simulink model "SpinningMode"  (R2024b)
settings: configuration reference "STM32H7_Config" (kept outside this file)
undefined symbols (not defined in the file): MSpin, nRPMSpinningModelIntegralActivation, NSpinningModelKi, NSpinningModelKp, nTargetRPM, tSpinLength, tTorqueControlTask
libraries: simulink x3, simulink_extras x1
settings Model: DataDictionary=Master_Dictionary.sldd  EnableAccessToBaseWorkspace=off  Creator=torni  LastModifiedBy=William
settings ConfigSetRef: SourceName=STM32H7_Config

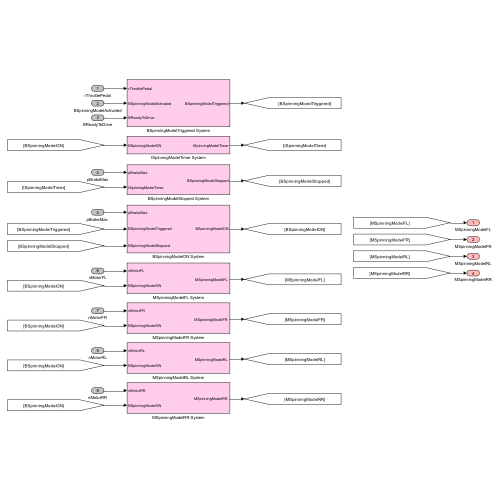
[thumbnail: Simulink's stored preview of the top-level diagram]
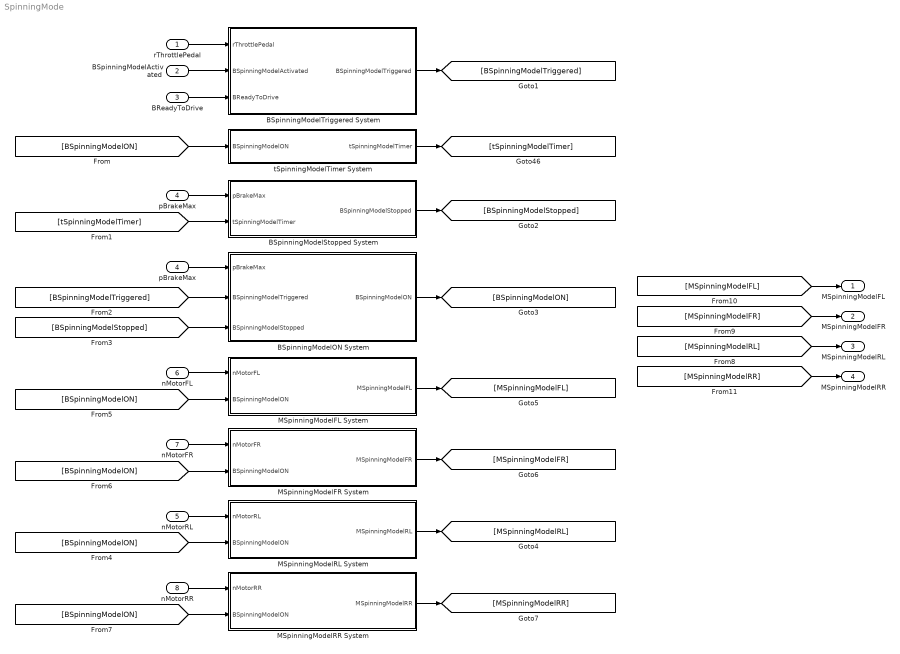
== system SpinningMode ==
  rThrottlePedal : Inport  OutDataTypeStr=double
  "BSpinningModelActivated " : Inport  Port=2  OutDataTypeStr=boolean
  BReadyToDrive : Inport  Port=3  OutDataTypeStr=boolean
  pBrakeMax : Inport  Port=4  OutDataTypeStr=double
  nMotorRL : Inport  Port=5  OutDataTypeStr=double
  nMotorFL : Inport  Port=6  OutDataTypeStr=double
  nMotorFR : Inport  Port=7  OutDataTypeStr=double
  nMotorRR : Inport  Port=8  OutDataTypeStr=double
  BSpinningModelON System : Subsystem
  BSpinningModelStopped System : Subsystem
  BSpinningModelTriggered System : Subsystem
  MSpinningModelFL System : Subsystem
  MSpinningModelFR System : Subsystem
  MSpinningModelRL System : Subsystem
  MSpinningModelRR System : Subsystem
  "pBrakeMax " : InportShadow  Port=4  OutDataTypeStr=double
  tSpinningModelTimer System : Subsystem
  MSpinningModelFL : Outport  OutDataTypeStr=double  VectorParamsAs1DForOutWhenUnconnected=off
  MSpinningModelFR : Outport  Port=2  OutDataTypeStr=double  VectorParamsAs1DForOutWhenUnconnected=off
  MSpinningModelRL : Outport  Port=3  OutDataTypeStr=double  VectorParamsAs1DForOutWhenUnconnected=off
  MSpinningModelRR : Outport  Port=4  OutDataTypeStr=double  VectorParamsAs1DForOutWhenUnconnected=off
  wires:
  rThrottlePedal/1 -> BSpinningModelTriggered System/1(rThrottlePedal)
  "BSpinningModelActivated "/1 -> BSpinningModelTriggered System/2("BSpinningModelActivated ")
  BReadyToDrive/1 -> BSpinningModelTriggered System/3(BReadyToDrive)
  pBrakeMax/1 -> BSpinningModelStopped System/1(pBrakeMax)
  [tSpinningModelTimer] -> BSpinningModelStopped System/2(tSpinningModelTimer)
  tSpinningModelTimer System/1(tSpinningModelTimer) -> [tSpinningModelTimer]
  BSpinningModelTriggered System/1(BSpinningModelTriggered) -> [BSpinningModelTriggered]
  BSpinningModelStopped System/1(BSpinningModelStopped) -> [BSpinningModelStopped]
  "pBrakeMax "/1 -> BSpinningModelON System/1(pBrakeMax)
  [BSpinningModelTriggered] -> BSpinningModelON System/2(BSpinningModelTriggered)
  [BSpinningModelStopped] -> BSpinningModelON System/3(BSpinningModelStopped)
  BSpinningModelON System/1(BSpinningModelON) -> [BSpinningModelON]
  [BSpinningModelON] -> tSpinningModelTimer System/1(BSpinningModelON)
  nMotorRL/1 -> MSpinningModelRL System/1(nMotorRL)
  [BSpinningModelON] -> MSpinningModelRL System/2(BSpinningModelON)
  MSpinningModelRL System/1("MSpinningModelRL ") -> [MSpinningModelRL]
  MSpinningModelFL System/1("MSpinningModelFL ") -> [MSpinningModelFL]
  [BSpinningModelON] -> MSpinningModelFL System/2(BSpinningModelON)
  nMotorFL/1 -> MSpinningModelFL System/1(nMotorFL)
  nMotorFR/1 -> MSpinningModelFR System/1(nMotorFR)
  [BSpinningModelON] -> MSpinningModelFR System/2(BSpinningModelON)
  MSpinningModelFR System/1("MSpinningModelFR ") -> [MSpinningModelFR]
  MSpinningModelRR System/1("MSpinningModelRR ") -> [MSpinningModelRR]
  [BSpinningModelON] -> MSpinningModelRR System/2(BSpinningModelON)
  nMotorRR/1 -> MSpinningModelRR System/1(nMotorRR)
  [MSpinningModelFL] -> MSpinningModelFL/1
  [MSpinningModelFR] -> MSpinningModelFR/1
  [MSpinningModelRR] -> MSpinningModelRR/1
  [MSpinningModelRL] -> MSpinningModelRL/1

== system SpinningMode/BSpinningModelON System ==
  pBrakeMax : Inport  OutDataTypeStr=double
  BSpinningModelTriggered : Inport  Port=2  OutDataTypeStr=boolean
  BSpinningModelStopped : Inport  Port=3  OutDataTypeStr=boolean
  Constant8 : Constant  Value=0
  S-R Flip-Flop : simulink_extras/Flip Flops/S-R Flip-Flop  initial_condition=0
  Switch3 : Switch  Criteria=u2 > Threshold  Threshold=1  SaturateOnIntegerOverflow=off  InputSameDT=off
  Terminator : Terminator
  BSpinningModelON : Outport  OutDataTypeStr=boolean  VectorParamsAs1DForOutWhenUnconnected=off
  wires:
  Switch3/1 -> BSpinningModelON/1
  BSpinningModelTriggered/1 -> S-R Flip-Flop/1
  Constant8/1 -> Switch3/1
  S-R Flip-Flop/1 -> Switch3/3
  S-R Flip-Flop/2 -> Terminator/1
  BSpinningModelStopped/1 -> S-R Flip-Flop/2
  pBrakeMax/1 -> Switch3/2

== system SpinningMode/BSpinningModelStopped System ==
  pBrakeMax : Inport  OutDataTypeStr=double
  tSpinningModelTimer : Inport  Port=2  OutDataTypeStr=double
  Compare To Constant : simulink/Logic and Bit Operations/Compare To Constant  relop=>  const=1  OutDataTypeStr=boolean
  Compare To Constant1 : simulink/Logic and Bit Operations/Compare To Constant  relop=>  const=tSpinLength  OutDataTypeStr=boolean
  OR1 : Logic  Operator=OR  AllPortsSameDT=off  OutDataTypeStr=boolean
  BSpinningModelStopped : Outport  OutDataTypeStr=boolean  VectorParamsAs1DForOutWhenUnconnected=off
  wires:
  Compare To Constant1/1 -> OR1/1
  Compare To Constant/1 -> OR1/2
  OR1/1 -> BSpinningModelStopped/1
  pBrakeMax/1 -> Compare To Constant/1
  tSpinningModelTimer/1 -> Compare To Constant1/1

== system SpinningMode/BSpinningModelTriggered System ==
  rThrottlePedal : Inport  OutDataTypeStr=double
  "BSpinningModelActivated " : Inport  Port=2  OutDataTypeStr=boolean
  BReadyToDrive : Inport  Port=3  OutDataTypeStr=boolean
  Compare To Constant : simulink/Logic and Bit Operations/Compare To Constant  relop=>  const=90  OutDataTypeStr=boolean
  Logical Operator : Logic  Inputs=3  AllPortsSameDT=off  OutDataTypeStr=boolean
  BSpinningModelTriggered : Outport  OutDataTypeStr=boolean  VectorParamsAs1DForOutWhenUnconnected=off
  wires:
  Logical Operator/1 -> BSpinningModelTriggered/1
  "BSpinningModelActivated "/1 -> Logical Operator/2
  rThrottlePedal/1 -> Compare To Constant/1
  Compare To Constant/1 -> Logical Operator/1
  BReadyToDrive/1 -> Logical Operator/3

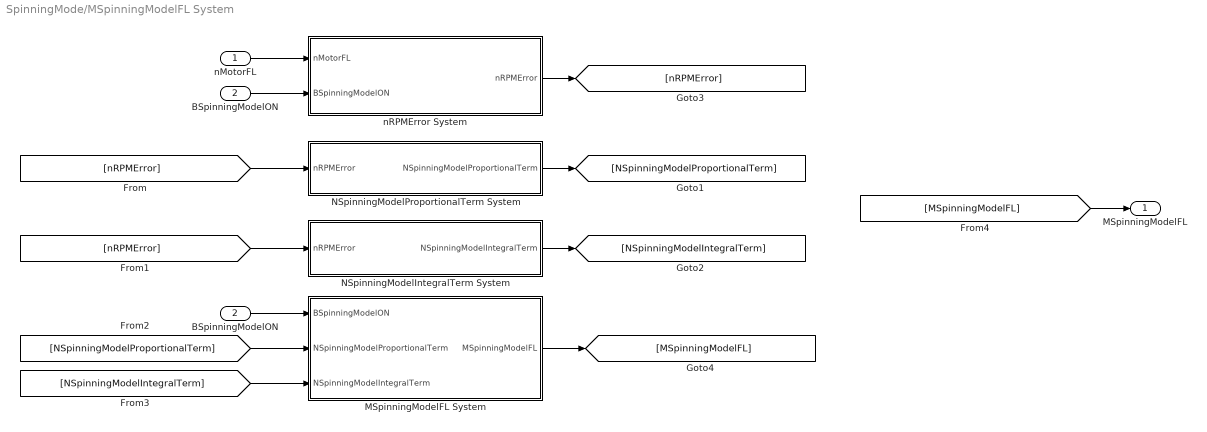
== system SpinningMode/MSpinningModelFL System ==
  nMotorFL : Inport  OutDataTypeStr=double
  BSpinningModelON : Inport  Port=2  OutDataTypeStr=boolean
  "BSpinningModelON " : InportShadow  Port=2  OutDataTypeStr=boolean
  MSpinningModelFL System : Subsystem
  NSpinningModelIntegralTerm System : Subsystem
  NSpinningModelProportionalTerm System : Subsystem
  nRPMError System : Subsystem
  "MSpinningModelFL " : Outport  OutDataTypeStr=double  VectorParamsAs1DForOutWhenUnconnected=off
  wires:
  [MSpinningModelFL] -> "MSpinningModelFL "/1
  MSpinningModelFL System/1("MSpinningModelFL ") -> [MSpinningModelFL]
  "BSpinningModelON "/1 -> MSpinningModelFL System/1(BSpinningModelON)
  [NSpinningModelIntegralTerm] -> MSpinningModelFL System/3(NSpinningModelIntegralTerm)
  [NSpinningModelProportionalTerm] -> MSpinningModelFL System/2(NSpinningModelProportionalTerm)
  NSpinningModelIntegralTerm System/1(NSpinningModelIntegralTerm) -> [NSpinningModelIntegralTerm]
  [nRPMError] -> NSpinningModelIntegralTerm System/1(nRPMError)
  NSpinningModelProportionalTerm System/1(NSpinningModelProportionalTerm) -> [NSpinningModelProportionalTerm]
  [nRPMError] -> NSpinningModelProportionalTerm System/1(nRPMError)
  nRPMError System/1(nRPMError) -> [nRPMError]
  BSpinningModelON/1 -> nRPMError System/2(BSpinningModelON)
  nMotorFL/1 -> nRPMError System/1(nMotorFL)

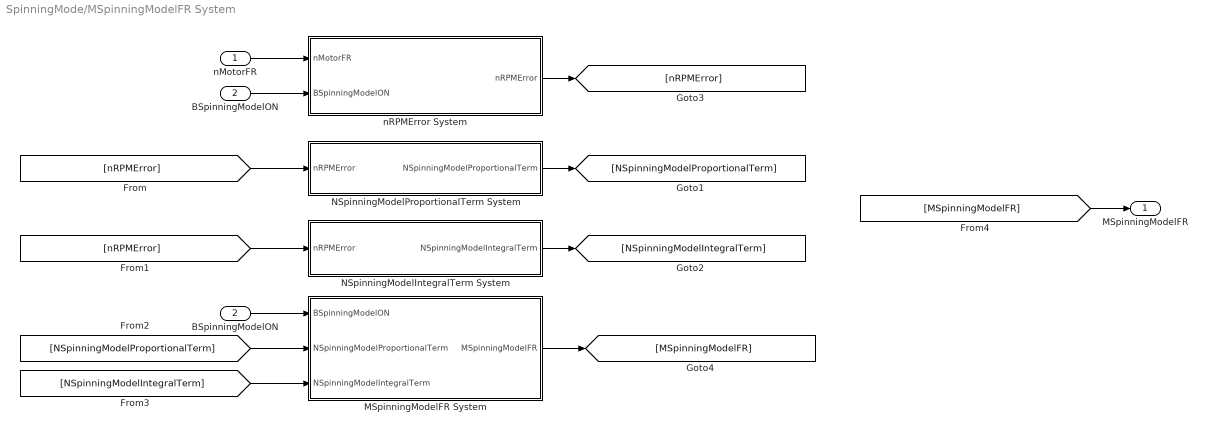
== system SpinningMode/MSpinningModelFR System ==
  nMotorFR : Inport  OutDataTypeStr=double
  BSpinningModelON : Inport  Port=2  OutDataTypeStr=boolean
  "BSpinningModelON " : InportShadow  Port=2  OutDataTypeStr=boolean
  MSpinningModelFR System : Subsystem
  NSpinningModelIntegralTerm System : Subsystem
  NSpinningModelProportionalTerm System : Subsystem
  nRPMError System : Subsystem
  "MSpinningModelFR " : Outport  OutDataTypeStr=double  VectorParamsAs1DForOutWhenUnconnected=off
  wires:
  nMotorFR/1 -> nRPMError System/1(nMotorFR)
  BSpinningModelON/1 -> nRPMError System/2(BSpinningModelON)
  nRPMError System/1(nRPMError) -> [nRPMError]
  [nRPMError] -> NSpinningModelProportionalTerm System/1(nRPMError)
  NSpinningModelProportionalTerm System/1(NSpinningModelProportionalTerm) -> [NSpinningModelProportionalTerm]
  [nRPMError] -> NSpinningModelIntegralTerm System/1(nRPMError)
  NSpinningModelIntegralTerm System/1(NSpinningModelIntegralTerm) -> [NSpinningModelIntegralTerm]
  [NSpinningModelProportionalTerm] -> MSpinningModelFR System/2(NSpinningModelProportionalTerm)
  [NSpinningModelIntegralTerm] -> MSpinningModelFR System/3(NSpinningModelIntegralTerm)
  "BSpinningModelON "/1 -> MSpinningModelFR System/1(BSpinningModelON)
  MSpinningModelFR System/1("MSpinningModelFR ") -> [MSpinningModelFR]
  [MSpinningModelFR] -> "MSpinningModelFR "/1

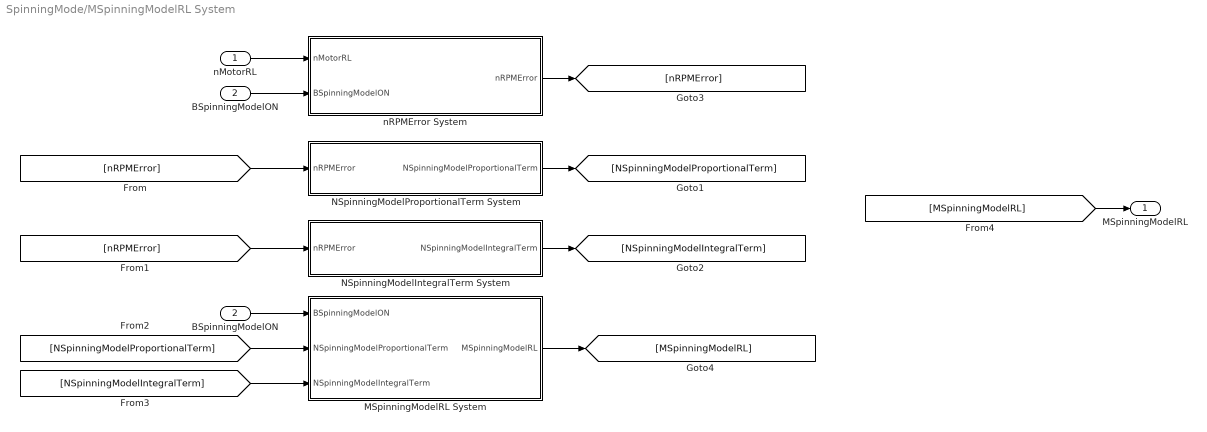
== system SpinningMode/MSpinningModelRL System ==
  nMotorRL : Inport  OutDataTypeStr=double
  BSpinningModelON : Inport  Port=2  OutDataTypeStr=boolean
  "BSpinningModelON " : InportShadow  Port=2  OutDataTypeStr=boolean
  MSpinningModelRL System : Subsystem
  NSpinningModelIntegralTerm System : Subsystem
  NSpinningModelProportionalTerm System : Subsystem
  nRPMError System : Subsystem
  "MSpinningModelRL " : Outport  OutDataTypeStr=double  VectorParamsAs1DForOutWhenUnconnected=off
  wires:
  nMotorRL/1 -> nRPMError System/1(nMotorRL)
  BSpinningModelON/1 -> nRPMError System/2(BSpinningModelON)
  nRPMError System/1(nRPMError) -> [nRPMError]
  [nRPMError] -> NSpinningModelProportionalTerm System/1(nRPMError)
  NSpinningModelProportionalTerm System/1(NSpinningModelProportionalTerm) -> [NSpinningModelProportionalTerm]
  [nRPMError] -> NSpinningModelIntegralTerm System/1(nRPMError)
  NSpinningModelIntegralTerm System/1(NSpinningModelIntegralTerm) -> [NSpinningModelIntegralTerm]
  [NSpinningModelProportionalTerm] -> MSpinningModelRL System/2(NSpinningModelProportionalTerm)
  [NSpinningModelIntegralTerm] -> MSpinningModelRL System/3(NSpinningModelIntegralTerm)
  "BSpinningModelON "/1 -> MSpinningModelRL System/1(BSpinningModelON)
  MSpinningModelRL System/1("MSpinningModelRL ") -> [MSpinningModelRL]
  [MSpinningModelRL] -> "MSpinningModelRL "/1

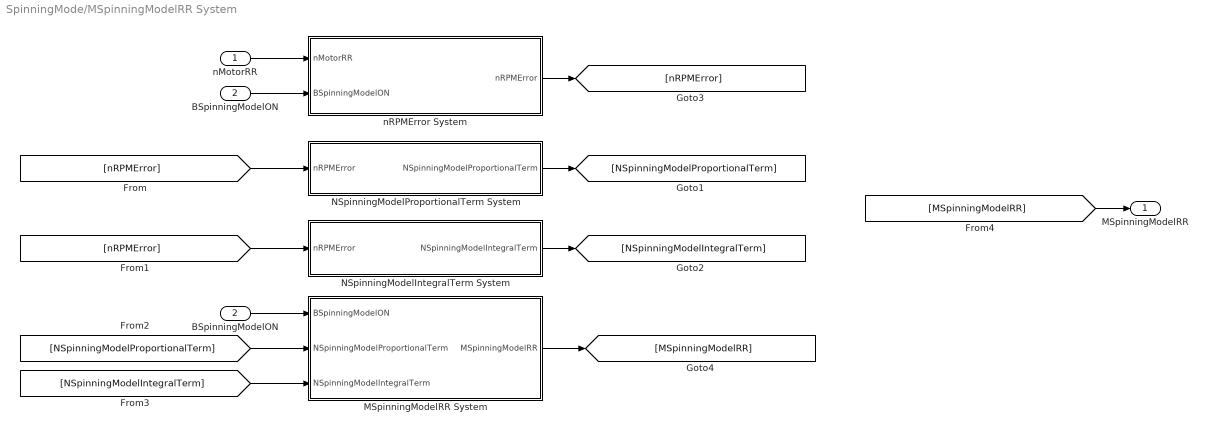
== system SpinningMode/MSpinningModelRR System ==
  nMotorRR : Inport  OutDataTypeStr=double
  BSpinningModelON : Inport  Port=2  OutDataTypeStr=boolean
  "BSpinningModelON " : InportShadow  Port=2  OutDataTypeStr=boolean
  MSpinningModelRR System : Subsystem
  NSpinningModelIntegralTerm System : Subsystem
  NSpinningModelProportionalTerm System : Subsystem
  nRPMError System : Subsystem
  "MSpinningModelRR " : Outport  OutDataTypeStr=double  VectorParamsAs1DForOutWhenUnconnected=off
  wires:
  [MSpinningModelRR] -> "MSpinningModelRR "/1
  MSpinningModelRR System/1("MSpinningModelRR ") -> [MSpinningModelRR]
  "BSpinningModelON "/1 -> MSpinningModelRR System/1(BSpinningModelON)
  [NSpinningModelIntegralTerm] -> MSpinningModelRR System/3(NSpinningModelIntegralTerm)
  [NSpinningModelProportionalTerm] -> MSpinningModelRR System/2(NSpinningModelProportionalTerm)
  NSpinningModelIntegralTerm System/1(NSpinningModelIntegralTerm) -> [NSpinningModelIntegralTerm]
  [nRPMError] -> NSpinningModelIntegralTerm System/1(nRPMError)
  NSpinningModelProportionalTerm System/1(NSpinningModelProportionalTerm) -> [NSpinningModelProportionalTerm]
  [nRPMError] -> NSpinningModelProportionalTerm System/1(nRPMError)
  nRPMError System/1(nRPMError) -> [nRPMError]
  BSpinningModelON/1 -> nRPMError System/2(BSpinningModelON)
  nMotorRR/1 -> nRPMError System/1(nMotorRR)

== system SpinningMode/tSpinningModelTimer System ==
  BSpinningModelON : Inport  OutDataTypeStr=boolean
  Add1 : Sum
  Constant5 : Constant  Value=tTorqueControlTask
  Constant6 : Constant  Value=0
  Memory1 : Memory  InheritSampleTime=on
  Switch1 : Switch  Criteria=u2 > Threshold  Threshold=0.5  SaturateOnIntegerOverflow=off  InputSameDT=off
  tSpinningModelTimer : Outport  OutDataTypeStr=double  VectorParamsAs1DForOutWhenUnconnected=off
  wires:
  Add1/1 -> Memory1/1
  Memory1/1 -> tSpinningModelTimer/1, Switch1/1
  Switch1/1 -> Add1/1
  Constant5/1 -> Add1/2
  Constant6/1 -> Switch1/3
  BSpinningModelON/1 -> Switch1/2

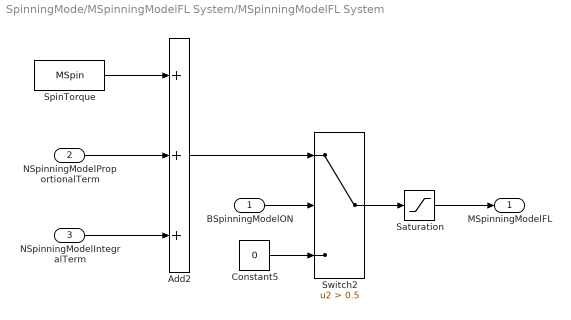
== system SpinningMode/MSpinningModelFL System/MSpinningModelFL System ==
  BSpinningModelON : Inport  OutDataTypeStr=boolean
  NSpinningModelProportionalTerm : Inport  Port=2  OutDataTypeStr=double
  NSpinningModelIntegralTerm : Inport  Port=3  OutDataTypeStr=double
  Add2 : Sum  Inputs=+++
  Constant5 : Constant  Value=0
  Saturation : Saturate  UpperLimit=13  LowerLimit=0
  SpinTorque : Constant  Value=MSpin
  Switch2 : Switch  Criteria=u2 > Threshold  Threshold=0.5  SaturateOnIntegerOverflow=off  InputSameDT=off
  "MSpinningModelFL " : Outport  OutDataTypeStr=double  VectorParamsAs1DForOutWhenUnconnected=off
  wires:
  NSpinningModelIntegralTerm/1 -> Add2/3
  NSpinningModelProportionalTerm/1 -> Add2/2
  Saturation/1 -> "MSpinningModelFL "/1
  Add2/1 -> Switch2/1
  BSpinningModelON/1 -> Switch2/2
  Constant5/1 -> Switch2/3
  SpinTorque/1 -> Add2/1
  Switch2/1 -> Saturation/1

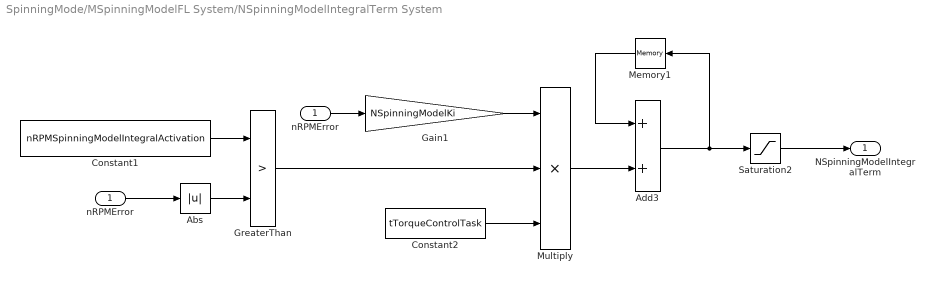
== system SpinningMode/MSpinningModelFL System/NSpinningModelIntegralTerm System ==
  nRPMError : Inport  OutDataTypeStr=double
  Abs : Abs  SaturateOnIntegerOverflow=off
  Add3 : Sum
  Constant1 : Constant  Value=nRPMSpinningModelIntegralActivation  VectorParams1D=off
  Constant2 : Constant  Value=tTorqueControlTask
  Gain1 : Gain  Gain=NSpinningModelKi
  GreaterThan : RelationalOperator  Operator=>  OutDataTypeStr=boolean  RndMeth=Simplest  InputSameDT=off
  Memory1 : Memory  InheritSampleTime=on
  Multiply : Product  Inputs=3
  Saturation2 : Saturate  UpperLimit=3  LowerLimit=-3
  "nRPMError " : InportShadow  OutDataTypeStr=double
  NSpinningModelIntegralTerm : Outport  OutDataTypeStr=double  VectorParamsAs1DForOutWhenUnconnected=off
  wires:
  Saturation2/1 -> NSpinningModelIntegralTerm/1
  Constant2/1 -> Multiply/3
  nRPMError/1 -> Abs/1
  GreaterThan/1 -> Multiply/2
  Abs/1 -> GreaterThan/2
  "nRPMError "/1 -> Gain1/1
  Multiply/1 -> Add3/2
  Constant1/1 -> GreaterThan/1
  Add3/1 -> Memory1/1, Saturation2/1
  Gain1/1 -> Multiply/1
  Memory1/1 -> Add3/1

== system SpinningMode/MSpinningModelFL System/NSpinningModelProportionalTerm System ==
  nRPMError : Inport  OutDataTypeStr=double
  Multiply1 : Product
  NSpinningModelKp : Lookup_n-D  NumberOfTableDimensions=1  BreakpointsForDimension1=[-3000, 0, 3000]  BreakpointsForDimension2=[1:3]  Table=[NSpinningModelKp, 0, NSpinningModelKp]  InternalRulePriority=Speed  RndMeth=Simplest
  Saturation1 : Saturate  UpperLimit=5  LowerLimit=-5
  "nRPMError " : InportShadow  OutDataTypeStr=double
  NSpinningModelProportionalTerm : Outport  OutDataTypeStr=double  VectorParamsAs1DForOutWhenUnconnected=off
  wires:
  Saturation1/1 -> NSpinningModelProportionalTerm/1
  "nRPMError "/1 -> Multiply1/2
  Multiply1/1 -> Saturation1/1
  NSpinningModelKp/1 -> Multiply1/1
  nRPMError/1 -> NSpinningModelKp/1

== system SpinningMode/MSpinningModelFL System/nRPMError System ==
  nMotorFL : Inport  OutDataTypeStr=double
  BSpinningModelON : Inport  Port=2  OutDataTypeStr=boolean
  Add1 : Sum  Inputs=+-
  Constant3 : Constant  Value=nTargetRPM
  Constant7 : Constant  Value=0
  Switch1 : Switch  Criteria=u2 > Threshold  Threshold=0.5  SaturateOnIntegerOverflow=off  InputSameDT=off
  nRPMError : Outport  OutDataTypeStr=double  VectorParamsAs1DForOutWhenUnconnected=off
  wires:
  Switch1/1 -> Add1/1
  nMotorFL/1 -> Add1/2
  Constant7/1 -> Switch1/3
  Constant3/1 -> Switch1/1
  Add1/1 -> nRPMError/1
  BSpinningModelON/1 -> Switch1/2

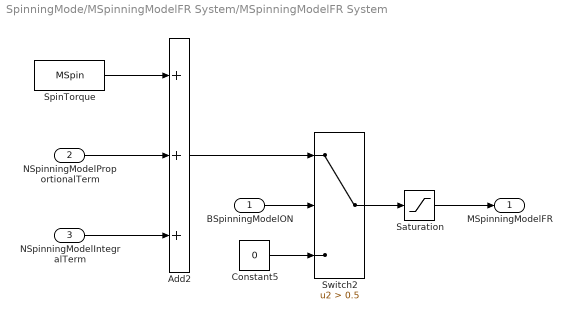
== system SpinningMode/MSpinningModelFR System/MSpinningModelFR System ==
  BSpinningModelON : Inport  OutDataTypeStr=boolean
  NSpinningModelProportionalTerm : Inport  Port=2  OutDataTypeStr=double
  NSpinningModelIntegralTerm : Inport  Port=3  OutDataTypeStr=double
  Add2 : Sum  Inputs=+++
  Constant5 : Constant  Value=0
  Saturation : Saturate  UpperLimit=13  LowerLimit=0
  SpinTorque : Constant  Value=MSpin
  Switch2 : Switch  Criteria=u2 > Threshold  Threshold=0.5  SaturateOnIntegerOverflow=off  InputSameDT=off
  "MSpinningModelFR " : Outport  OutDataTypeStr=double  VectorParamsAs1DForOutWhenUnconnected=off
  wires:
  Switch2/1 -> Saturation/1
  SpinTorque/1 -> Add2/1
  Constant5/1 -> Switch2/3
  BSpinningModelON/1 -> Switch2/2
  Add2/1 -> Switch2/1
  Saturation/1 -> "MSpinningModelFR "/1
  NSpinningModelProportionalTerm/1 -> Add2/2
  NSpinningModelIntegralTerm/1 -> Add2/3

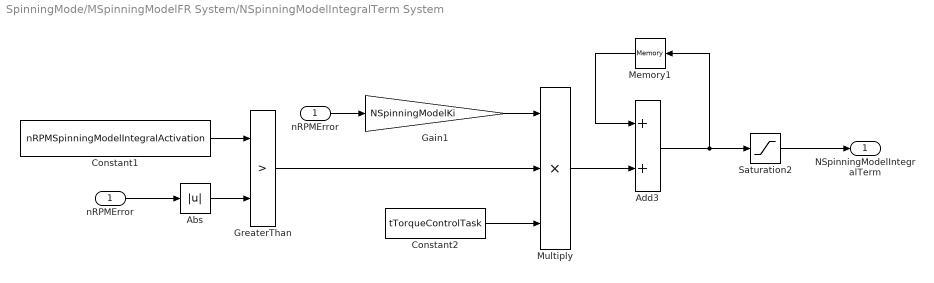
== system SpinningMode/MSpinningModelFR System/NSpinningModelIntegralTerm System ==
  nRPMError : Inport  OutDataTypeStr=double
  Abs : Abs  SaturateOnIntegerOverflow=off
  Add3 : Sum
  Constant1 : Constant  Value=nRPMSpinningModelIntegralActivation  VectorParams1D=off
  Constant2 : Constant  Value=tTorqueControlTask
  Gain1 : Gain  Gain=NSpinningModelKi
  GreaterThan : RelationalOperator  Operator=>  OutDataTypeStr=boolean  RndMeth=Simplest  InputSameDT=off
  Memory1 : Memory  InheritSampleTime=on
  Multiply : Product  Inputs=3
  Saturation2 : Saturate  UpperLimit=3  LowerLimit=-3
  "nRPMError " : InportShadow  OutDataTypeStr=double
  NSpinningModelIntegralTerm : Outport  OutDataTypeStr=double  VectorParamsAs1DForOutWhenUnconnected=off
  wires:
  Memory1/1 -> Add3/1
  Gain1/1 -> Multiply/1
  Add3/1 -> Saturation2/1, Memory1/1
  Constant1/1 -> GreaterThan/1
  Multiply/1 -> Add3/2
  "nRPMError "/1 -> Gain1/1
  Abs/1 -> GreaterThan/2
  GreaterThan/1 -> Multiply/2
  nRPMError/1 -> Abs/1
  Constant2/1 -> Multiply/3
  Saturation2/1 -> NSpinningModelIntegralTerm/1

== system SpinningMode/MSpinningModelFR System/NSpinningModelProportionalTerm System ==
  nRPMError : Inport  OutDataTypeStr=double
  Multiply1 : Product
  NSpinningModelKp : Lookup_n-D  NumberOfTableDimensions=1  BreakpointsForDimension1=[-3000, 0, 3000]  BreakpointsForDimension2=[1:3]  Table=[NSpinningModelKp, 0, NSpinningModelKp]  InternalRulePriority=Speed  RndMeth=Simplest
  Saturation1 : Saturate  UpperLimit=5  LowerLimit=-5
  "nRPMError " : InportShadow  OutDataTypeStr=double
  NSpinningModelProportionalTerm : Outport  OutDataTypeStr=double  VectorParamsAs1DForOutWhenUnconnected=off
  wires:
  nRPMError/1 -> NSpinningModelKp/1
  NSpinningModelKp/1 -> Multiply1/1
  Multiply1/1 -> Saturation1/1
  "nRPMError "/1 -> Multiply1/2
  Saturation1/1 -> NSpinningModelProportionalTerm/1

== system SpinningMode/MSpinningModelFR System/nRPMError System ==
  nMotorFR : Inport  OutDataTypeStr=double
  BSpinningModelON : Inport  Port=2  OutDataTypeStr=boolean
  Add1 : Sum  Inputs=+-
  Constant3 : Constant  Value=nTargetRPM
  Constant7 : Constant  Value=0
  Switch1 : Switch  Criteria=u2 > Threshold  Threshold=0.5  SaturateOnIntegerOverflow=off  InputSameDT=off
  nRPMError : Outport  OutDataTypeStr=double  VectorParamsAs1DForOutWhenUnconnected=off
  wires:
  BSpinningModelON/1 -> Switch1/2
  Add1/1 -> nRPMError/1
  Constant3/1 -> Switch1/1
  Constant7/1 -> Switch1/3
  nMotorFR/1 -> Add1/2
  Switch1/1 -> Add1/1

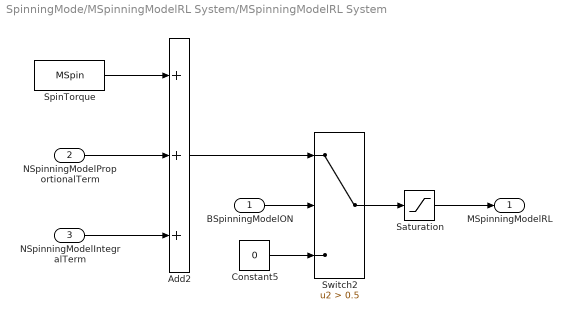
== system SpinningMode/MSpinningModelRL System/MSpinningModelRL System ==
  BSpinningModelON : Inport  OutDataTypeStr=boolean
  NSpinningModelProportionalTerm : Inport  Port=2  OutDataTypeStr=double
  NSpinningModelIntegralTerm : Inport  Port=3  OutDataTypeStr=double
  Add2 : Sum  Inputs=+++
  Constant5 : Constant  Value=0
  Saturation : Saturate  UpperLimit=13  LowerLimit=0
  SpinTorque : Constant  Value=MSpin
  Switch2 : Switch  Criteria=u2 > Threshold  Threshold=0.5  SaturateOnIntegerOverflow=off  InputSameDT=off
  "MSpinningModelRL " : Outport  OutDataTypeStr=double  VectorParamsAs1DForOutWhenUnconnected=off
  wires:
  Switch2/1 -> Saturation/1
  SpinTorque/1 -> Add2/1
  Constant5/1 -> Switch2/3
  BSpinningModelON/1 -> Switch2/2
  Add2/1 -> Switch2/1
  Saturation/1 -> "MSpinningModelRL "/1
  NSpinningModelProportionalTerm/1 -> Add2/2
  NSpinningModelIntegralTerm/1 -> Add2/3

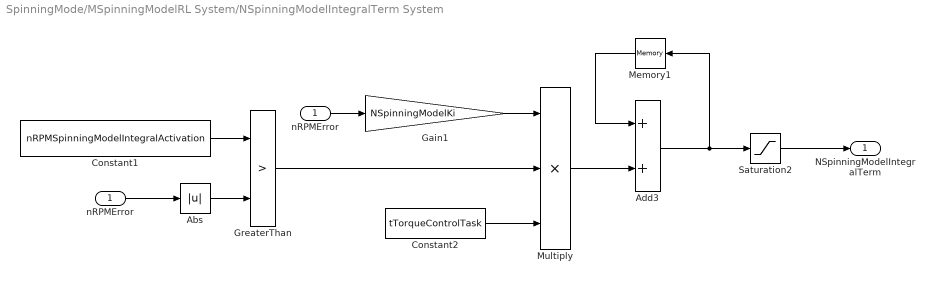
== system SpinningMode/MSpinningModelRL System/NSpinningModelIntegralTerm System ==
  nRPMError : Inport  OutDataTypeStr=double
  Abs : Abs  SaturateOnIntegerOverflow=off
  Add3 : Sum
  Constant1 : Constant  Value=nRPMSpinningModelIntegralActivation  VectorParams1D=off
  Constant2 : Constant  Value=tTorqueControlTask
  Gain1 : Gain  Gain=NSpinningModelKi
  GreaterThan : RelationalOperator  Operator=>  OutDataTypeStr=boolean  RndMeth=Simplest  InputSameDT=off
  Memory1 : Memory  InheritSampleTime=on
  Multiply : Product  Inputs=3
  Saturation2 : Saturate  UpperLimit=3  LowerLimit=-3
  "nRPMError " : InportShadow  OutDataTypeStr=double
  NSpinningModelIntegralTerm : Outport  OutDataTypeStr=double  VectorParamsAs1DForOutWhenUnconnected=off
  wires:
  Memory1/1 -> Add3/1
  Gain1/1 -> Multiply/1
  Add3/1 -> Saturation2/1, Memory1/1
  Constant1/1 -> GreaterThan/1
  Multiply/1 -> Add3/2
  "nRPMError "/1 -> Gain1/1
  Abs/1 -> GreaterThan/2
  GreaterThan/1 -> Multiply/2
  nRPMError/1 -> Abs/1
  Constant2/1 -> Multiply/3
  Saturation2/1 -> NSpinningModelIntegralTerm/1

== system SpinningMode/MSpinningModelRL System/NSpinningModelProportionalTerm System ==
  nRPMError : Inport  OutDataTypeStr=double
  Multiply1 : Product
  NSpinningModelKp : Lookup_n-D  NumberOfTableDimensions=1  BreakpointsForDimension1=[-3000, 0, 3000]  BreakpointsForDimension2=[1:3]  Table=[NSpinningModelKp, 0, NSpinningModelKp]  InternalRulePriority=Speed  RndMeth=Simplest
  Saturation1 : Saturate  UpperLimit=5  LowerLimit=-5
  "nRPMError " : InportShadow  OutDataTypeStr=double
  NSpinningModelProportionalTerm : Outport  OutDataTypeStr=double  VectorParamsAs1DForOutWhenUnconnected=off
  wires:
  nRPMError/1 -> NSpinningModelKp/1
  NSpinningModelKp/1 -> Multiply1/1
  Multiply1/1 -> Saturation1/1
  "nRPMError "/1 -> Multiply1/2
  Saturation1/1 -> NSpinningModelProportionalTerm/1

== system SpinningMode/MSpinningModelRL System/nRPMError System ==
  nMotorRL : Inport  OutDataTypeStr=double
  BSpinningModelON : Inport  Port=2  OutDataTypeStr=boolean
  Add1 : Sum  Inputs=+-
  Constant3 : Constant  Value=nTargetRPM
  Constant7 : Constant  Value=0
  Switch1 : Switch  Criteria=u2 > Threshold  Threshold=0.5  SaturateOnIntegerOverflow=off  InputSameDT=off
  nRPMError : Outport  OutDataTypeStr=double  VectorParamsAs1DForOutWhenUnconnected=off
  wires:
  BSpinningModelON/1 -> Switch1/2
  Add1/1 -> nRPMError/1
  Constant3/1 -> Switch1/1
  Constant7/1 -> Switch1/3
  nMotorRL/1 -> Add1/2
  Switch1/1 -> Add1/1

== system SpinningMode/MSpinningModelRR System/MSpinningModelRR System ==
  BSpinningModelON : Inport  OutDataTypeStr=boolean
  NSpinningModelProportionalTerm : Inport  Port=2  OutDataTypeStr=double
  NSpinningModelIntegralTerm : Inport  Port=3  OutDataTypeStr=double
  Add2 : Sum  Inputs=+++
  Constant5 : Constant  Value=0
  Saturation : Saturate  UpperLimit=13  LowerLimit=0
  SpinTorque : Constant  Value=MSpin
  Switch2 : Switch  Criteria=u2 > Threshold  Threshold=0.5  SaturateOnIntegerOverflow=off  InputSameDT=off
  "MSpinningModelRR " : Outport  OutDataTypeStr=double  VectorParamsAs1DForOutWhenUnconnected=off
  wires:
  NSpinningModelIntegralTerm/1 -> Add2/3
  NSpinningModelProportionalTerm/1 -> Add2/2
  Saturation/1 -> "MSpinningModelRR "/1
  Add2/1 -> Switch2/1
  BSpinningModelON/1 -> Switch2/2
  Constant5/1 -> Switch2/3
  SpinTorque/1 -> Add2/1
  Switch2/1 -> Saturation/1

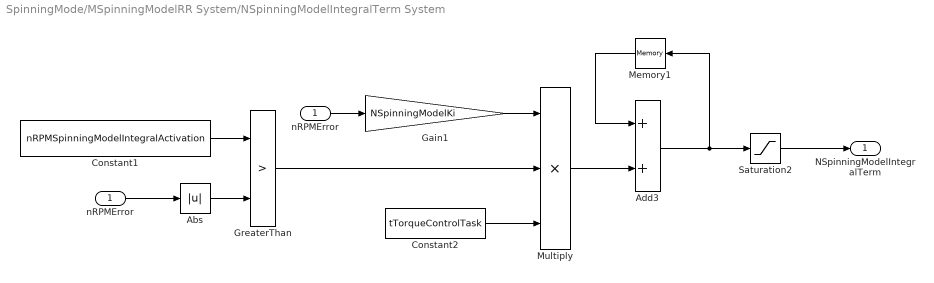
== system SpinningMode/MSpinningModelRR System/NSpinningModelIntegralTerm System ==
  nRPMError : Inport  OutDataTypeStr=double
  Abs : Abs  SaturateOnIntegerOverflow=off
  Add3 : Sum
  Constant1 : Constant  Value=nRPMSpinningModelIntegralActivation  VectorParams1D=off
  Constant2 : Constant  Value=tTorqueControlTask
  Gain1 : Gain  Gain=NSpinningModelKi
  GreaterThan : RelationalOperator  Operator=>  OutDataTypeStr=boolean  RndMeth=Simplest  InputSameDT=off
  Memory1 : Memory  InheritSampleTime=on
  Multiply : Product  Inputs=3
  Saturation2 : Saturate  UpperLimit=3  LowerLimit=-3
  "nRPMError " : InportShadow  OutDataTypeStr=double
  NSpinningModelIntegralTerm : Outport  OutDataTypeStr=double  VectorParamsAs1DForOutWhenUnconnected=off
  wires:
  Saturation2/1 -> NSpinningModelIntegralTerm/1
  Constant2/1 -> Multiply/3
  nRPMError/1 -> Abs/1
  GreaterThan/1 -> Multiply/2
  Abs/1 -> GreaterThan/2
  "nRPMError "/1 -> Gain1/1
  Multiply/1 -> Add3/2
  Constant1/1 -> GreaterThan/1
  Add3/1 -> Memory1/1, Saturation2/1
  Gain1/1 -> Multiply/1
  Memory1/1 -> Add3/1

== system SpinningMode/MSpinningModelRR System/NSpinningModelProportionalTerm System ==
  nRPMError : Inport  OutDataTypeStr=double
  Multiply1 : Product
  NSpinningModelKp : Lookup_n-D  NumberOfTableDimensions=1  BreakpointsForDimension1=[-3000, 0, 3000]  BreakpointsForDimension2=[1:3]  Table=[NSpinningModelKp, 0, NSpinningModelKp]  InternalRulePriority=Speed  RndMeth=Simplest
  Saturation1 : Saturate  UpperLimit=5  LowerLimit=-5
  "nRPMError " : InportShadow  OutDataTypeStr=double
  NSpinningModelProportionalTerm : Outport  OutDataTypeStr=double  VectorParamsAs1DForOutWhenUnconnected=off
  wires:
  Saturation1/1 -> NSpinningModelProportionalTerm/1
  "nRPMError "/1 -> Multiply1/2
  Multiply1/1 -> Saturation1/1
  NSpinningModelKp/1 -> Multiply1/1
  nRPMError/1 -> NSpinningModelKp/1

== system SpinningMode/MSpinningModelRR System/nRPMError System ==
  nMotorRR : Inport  OutDataTypeStr=double
  BSpinningModelON : Inport  Port=2  OutDataTypeStr=boolean
  Add1 : Sum  Inputs=+-
  Constant3 : Constant  Value=nTargetRPM
  Constant7 : Constant  Value=0
  Switch1 : Switch  Criteria=u2 > Threshold  Threshold=0.5  SaturateOnIntegerOverflow=off  InputSameDT=off
  nRPMError : Outport  OutDataTypeStr=double  VectorParamsAs1DForOutWhenUnconnected=off
  wires:
  Switch1/1 -> Add1/1
  nMotorRR/1 -> Add1/2
  Constant7/1 -> Switch1/3
  Constant3/1 -> Switch1/1
  Add1/1 -> nRPMError/1
  BSpinningModelON/1 -> Switch1/2
